simulink model "sim_olp_y"  (R2018a)
settings: Solver=ode3  StartTime=0.0  StopTime=10.0  FixedStep=0.01  RelTol=1e-3
values from neighbouring files (symbols this model uses):
  A = [-(Cf+Cr)/(m*Vx)  -(a*Cf-b*Cr)/(m*Vx)-Vx ... (first row only)    [lin_control_pos_v1.m]    (also in lin_control_y.m)
  B = [Cf/m; a*Cf/Iz]    [lin_control_pos_v1.m]    (also in lin_control_y.m)
  g = 9.81    [lin_control_pos_v1.m]    (also in lin_control_y.m)
  rho = 1/R    (= 0.05)    [lin_control_pos_v1.m]    (also in lin_control_y.m)
  Vx = 10/3.6    (= 2.77777777778)    [lin_control_pos_v1.m]    (also in lin_control_y.m)
  w = 10    [lin_control_pos_v1.m]    (also in lin_control_y.m)
settings Model: Creator=E183308  LastModifiedBy=E183308

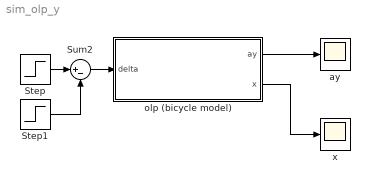
== system sim_olp_y ==
  Step : Step  After=10*pi/180  SampleTime=0
  Step1 : Step  Time=3  After=10*pi/180  SampleTime=0
  Sum2 : Sum  Inputs=|+-
  ay : Scope
  olp (bicycle model) : Subsystem
  x : Scope
  wires:
  Step1/1 -> Sum2/2
  Sum2/1 -> olp (bicycle model)/1(delta)
  Step/1 -> Sum2/1
  olp (bicycle model)/1(ay) -> ay/1
  olp (bicycle model)/2(x) -> x/1

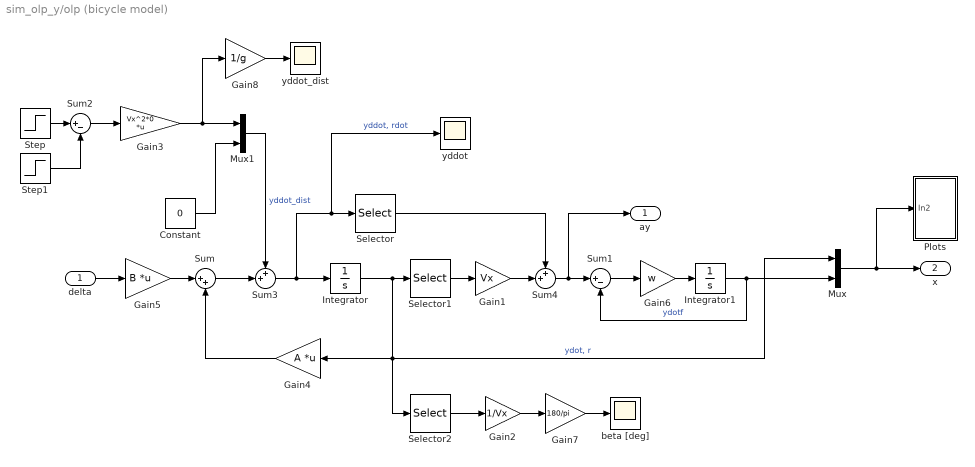
== system sim_olp_y/olp (bicycle model) ==
  delta : Inport
  Constant : Constant  Value=0
  Gain1 : Gain  Gain=Vx
  Gain2 : Gain  Gain=1/Vx
  Gain3 : Gain  Gain=Vx^2*0  Multiplication=Matrix(K*u)
  Gain4 : Gain  Gain=A  Multiplication=Matrix(K*u)
  Gain5 : Gain  Gain=B  Multiplication=Matrix(K*u)
  Gain6 : Gain  Gain=w
  Gain7 : Gain  Gain=180/pi
  Gain8 : Gain  Gain=1/g
  Integrator : Integrator  InitialCondition=[0;0]
  Integrator1 : Integrator
  Mux : Mux  Inputs=2
  Mux1 : Mux  Inputs=2
  Plots : Subsystem
  Selector : Selector  InputPortWidth=2  IndexOptions=Index vector (dialog)  Indices=1  OutputSizes=1
  Selector1 : Selector  InputPortWidth=2  IndexOptions=Index vector (dialog)  Indices=2  OutputSizes=1
  Selector2 : Selector  InputPortWidth=2  IndexOptions=Index vector (dialog)  Indices=1  OutputSizes=1
  Step : Step  After=rho  SampleTime=0
  Step1 : Step  Time=10  After=rho  SampleTime=0
  Sum : Sum  Inputs=|++
  Sum1 : Sum  Inputs=|+-
  Sum2 : Sum  Inputs=|+-
  Sum3 : Sum  Inputs=++|
  Sum4 : Sum  Inputs=++|
  beta [deg] : Scope
  yddot : Scope
  yddot_dist : Scope
  ay : Outport
  x : Outport  Port=2
  wires:
  Integrator/1 -> Selector1/1, Selector2/1, Gain4/1, Mux/1  "ydot, r"
  delta/1 -> Gain5/1
  Gain5/1 -> Sum/1
  Gain4/1 -> Sum/2
  Gain6/1 -> Integrator1/1
  Sum1/1 -> Gain6/1
  Mux/1 -> Plots/1(In2), x/1
  Integrator1/1 -> Sum1/2, Mux/2  "ydotf"
  Gain8/1 -> yddot_dist/1
  Sum2/1 -> Gain3/1
  Step/1 -> Sum2/1
  Step1/1 -> Sum2/2
  Sum/1 -> Sum3/2
  Sum3/1 -> yddot/1, Selector/1, Integrator/1  "yddot, rdot"
  Gain3/1 -> Mux1/1, Gain8/1
  Mux1/1 -> Sum3/1  "yddot_dist"
  Constant/1 -> Mux1/2
  Selector1/1 -> Gain1/1
  Gain1/1 -> Sum4/2
  Selector/1 -> Sum4/1
  Sum4/1 -> ay/1, Sum1/1
  Selector2/1 -> Gain2/1
  Gain2/1 -> Gain7/1
  Gain7/1 -> beta [deg]/1

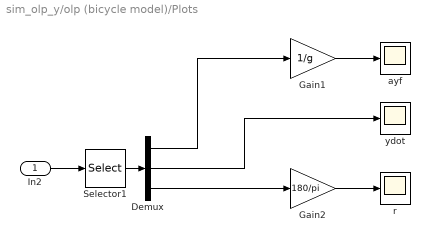
== system sim_olp_y/olp (bicycle model)/Plots ==
  In2 : Inport
  Demux : Demux  Outputs=3
  Gain1 : Gain  Gain=1/g
  Gain2 : Gain  Gain=180/pi
  Selector1 : Selector  InputPortWidth=3  IndexOptions=Index vector (dialog)  Indices=[3 1 2]  OutputSizes=1
  ayf : Scope
  r : Scope
  ydot : Scope
  wires:
  Demux/2 -> ydot/1
  Demux/3 -> Gain2/1
  Gain2/1 -> r/1
  In2/1 -> Selector1/1
  Demux/1 -> Gain1/1
  Selector1/1 -> Demux/1
  Gain1/1 -> ayf/1
